simulink model "inverted_pendulum"  (R2020a)
settings: Solver=FixedStepAuto  StartTime=0.0  StopTime=100  FixedStep=0.001  MaxStep=0.001  RelTol=1e-3
settings Model: Creator=chinm  LastModifiedBy=chinm

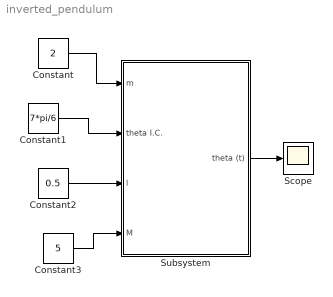
== system inverted_pendulum ==
  Constant : Constant  Value=2
  Constant1 : Constant  Value=7*pi/6
  Constant2 : Constant  Value=0.5
  Constant3 : Constant  Value=5
  Scope : Scope
  Subsystem : Subsystem
  wires:
  Constant1/1 -> Subsystem/2(theta I.C.)
  Constant/1 -> Subsystem/1(m)
  Constant2/1 -> Subsystem/3(l)
  Constant3/1 -> Subsystem/4(M)
  Subsystem/1(theta (t)) -> Scope/1

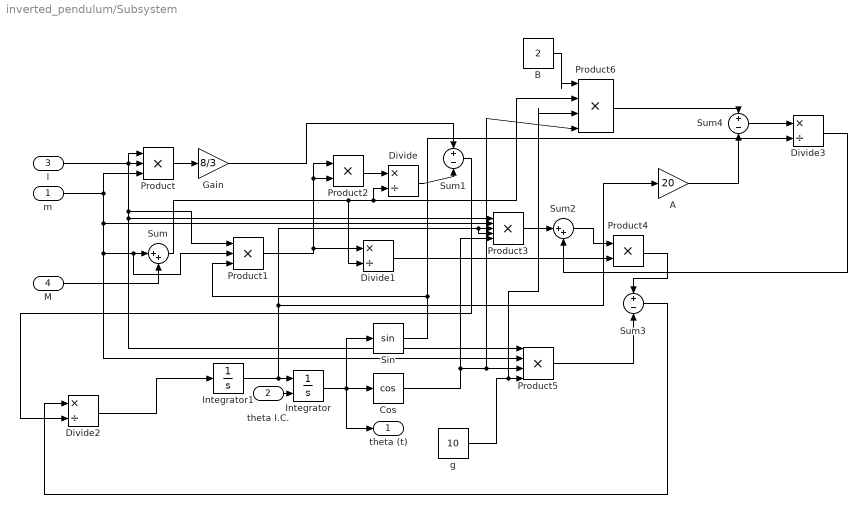
== system inverted_pendulum/Subsystem ==
  m : Inport
  theta I.C. : Inport  Port=2
  l : Inport  Port=3
  M : Inport  Port=4
  A : Gain  Gain=20
  B : Constant  Value=2
  Cos : Trigonometry  Operator=cos
  Divide{,1..3} (4 alike) : Product  Inputs=*/
  Gain : Gain  Gain=8/3
  Integrator : Integrator  InitialConditionSource=external
  Integrator1 : Integrator
  Product : Product  Inputs=3
  Product1 : Product  Inputs=3
  Product2 : Product
  Product3 : Product  Inputs=5
  Product4 : Product
  Product5 : Product  Inputs=4
  Product6 : Product  Inputs=4
  Sin : Trigonometry
  Sum : Sum  Inputs=|++
  Sum1 : Sum  Inputs=+-
  Sum2 : Sum  Inputs=|++
  Sum3 : Sum  Inputs=+-
  Sum4 : Sum  Inputs=+-
  g : Constant  Value=10
  theta (t) : Outport
  wires:
  theta I.C./1 -> Integrator/2
  Integrator1/1 -> A/1, Product3/4, Product3/3, Integrator/1
  m/1 -> Product5/2, Product1/2, Sum/1, Product3/2, Product/3
  l/1 -> Product/1, Product5/1, Product3/1, Product1/1, Product/2
  Product/1 -> Gain/1
  Integrator/1 -> Sin/1, theta (t)/1, Cos/1
  M/1 -> Sum/2
  Sin/1 -> Divide3/2, Product1/3
  Product1/1 -> Divide1/1, Product2/2, Product2/1
  Product2/1 -> Divide/1
  Sum/1 -> Divide/2, Product6/2, Divide1/2
  Gain/1 -> Sum1/1
  Divide/1 -> Sum1/2
  Cos/1 -> Product5/3, Product6/4, Product3/5
  Product3/1 -> Sum2/1
  Divide1/1 -> Product4/2
  Sum2/1 -> Product4/1
  g/1 -> Product6/3, Product5/4
  Product4/1 -> Sum3/1
  Product5/1 -> Sum3/2
  Sum3/1 -> Divide2/1
  Sum1/1 -> Divide2/2
  Divide2/1 -> Integrator1/1
  B/1 -> Product6/1
  Product6/1 -> Sum4/1
  Sum4/1 -> Divide3/1
  Divide3/1 -> Sum2/2
  A/1 -> Sum4/2
